simulink model "untitled"  (Simulink 7.9)
settings: Solver=ode45  StartTime=0.0  StopTime=10.0  RelTol=1e-3
settings Model: Creator=simena  LastModifiedBy=simena

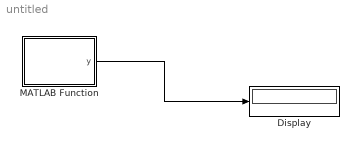
== system untitled ==
  Display : Display
  MATLAB Function : MATLAB Function  TreatAsAtomicUnit=on
  wires:
  MATLAB Function/1(y) -> Display/1

== matlab function MATLAB Function ==
  data: y output double
function y = fcn()
%#codegen
y= fcn2(2);

    

end

function a=fcn2(b)
       a=2*b; 
end
